simulink model "FINAL_APPROACH_CUSTOM"  (R2020b)
settings: Solver=ode5  StartTime=0.0  StopTime=10  FixedStep=0.01  RelTol=1e-3
values from neighbouring files (symbols this model uses):
  alpha = 0.01    [INPUTS_GRUPPO20.m]
  e_ss = 0.02    [INPUTS_GRUPPO20.m]
  enable_drag = 1    [INPUTS_GRUPPO20.m]
  enable_J2 = 1    [INPUTS_GRUPPO20.m]
  enable_Mgrav = 1    [INPUTS_GRUPPO20.m]
  enable_PD = 1    [INPUTS_GRUPPO20.m]
  enable_SMC = 0    [INPUTS_GRUPPO20.m]
  F_D = -1/2*rho*CD*A*Vx^2    (= -3.88125057814e-05)    [INPUTS_GRUPPO20.m]
  FJ2 = -3*J2*m_c0*mu*r_E^2/(2*r^4)    (= -0.00149705073945)    [INPUTS_GRUPPO20.m]
  gmax = 0.005    [INPUTS_GRUPPO20.m]
  INV_ZZZ = pinv(ZZZ)    [INPUTS_GRUPPO20.m]
  invJ = inv(J)    [INPUTS_GRUPPO20.m]
  Isp1 = 220    [INPUTS_GRUPPO20.m]
  J = J0    [INPUTS_GRUPPO20.m]
  kd = d*eye(3)    [INPUTS_GRUPPO20.m]
  Kd = [1 0.1 1]'    [INPUTS_GRUPPO20.m]
  kf = U_max/edb    (= 10)    [INPUTS_GRUPPO20.m]
  Kp = [0.00001 0.05 0.01]'    [INPUTS_GRUPPO20.m]
  kp1 = k*eye(3)    [INPUTS_GRUPPO20.m]
  Kr = 1    [INPUTS_GRUPPO20.m]
  lambda = 0.03    [INPUTS_GRUPPO20.m]
  m_c0_CUS = m_RB(end)    [INPUTS_GRUPPO20.m]
  omega = (mu/r^3)^0.5    (= 0.00113136572666)    [INPUTS_GRUPPO20.m]
  p_RW = 1    [INPUTS_GRUPPO20.m]
  Pos0 = Pos_RB(end,:)'    [INPUTS_GRUPPO20.m]
  q0_0 = Q_RB(end,1)'    [INPUTS_GRUPPO20.m]
  q_des = [1 0 0 0]'    [INPUTS_GRUPPO20.m]
  qv_0 = Q_RB(end,2:4)'    [INPUTS_GRUPPO20.m]
  tau = -deltaton/log((1-(U_on-U_off)/kf))    [INPUTS_GRUPPO20.m]
  tau_RW = 1.5645e-2    (= 0.015645)    [INPUTS_GRUPPO20.m]
  U_max = 2    [INPUTS_GRUPPO20.m]
  U_off = 0.29    [INPUTS_GRUPPO20.m]
  U_on = 1    [INPUTS_GRUPPO20.m]
  Vel0 = Vel_RB(end,:)'    [INPUTS_GRUPPO20.m]
  wb_0 = wb_RB(end,:)'    [INPUTS_GRUPPO20.m]
  ZZZ = [cos(B)    0      -cos(B)    0 ... (first row only)    [INPUTS_GRUPPO20.m]
undefined symbols (not defined in the file or in its folder): DiscIntNeverNeededParam, magnitude
libraries: vrlib x3, aerolibutil x1, sharedtransform x1
settings Model: Creator=Lucas  LastModifiedBy=Beniamino

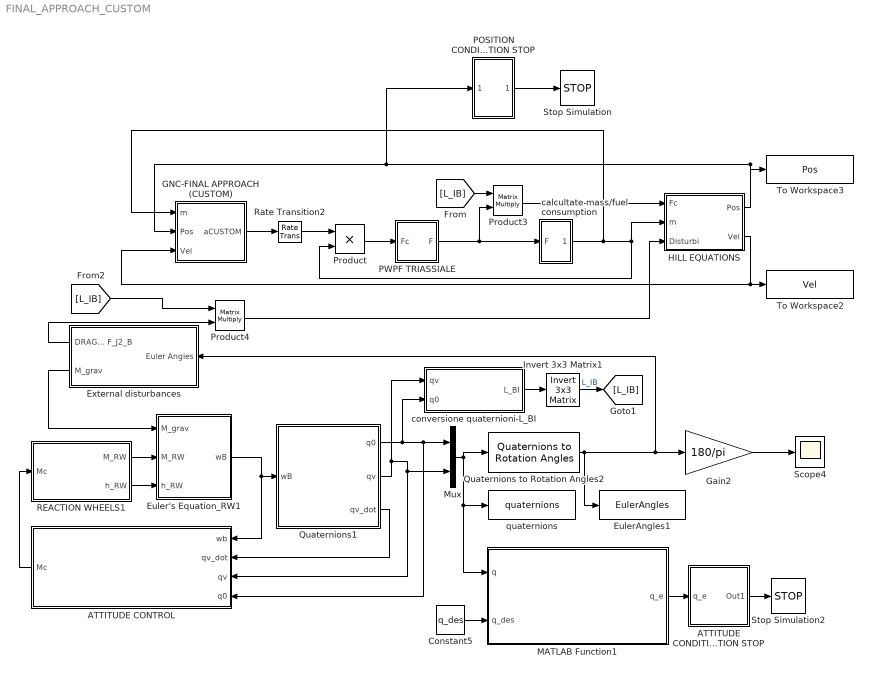
== system FINAL_APPROACH_CUSTOM ==
  ATTITUDE CONDITION SIMULATION STOP : Subsystem
  ATTITUDE CONTROL : Subsystem
  Constant5 : Constant  Value=q_des
  Euler's Equation_RW1 : Subsystem
  EulerAngles1 : ToWorkspace  VariableName=EulerAngles  SampleTime=-1
  External disturbances : Subsystem
  GNC-FINAL APPROACH (CUSTOM) : Subsystem
  Gain2 : Gain  Gain=180/pi
  HILL EQUATIONS : Subsystem
  Invert 3x3 Matrix1 : aerolibutil/Invert  3x3 Matrix
  MATLAB Function1 : MATLAB Function  TreatAsAtomicUnit=on
  Mux : Mux  Inputs=2
  POSITION CONDITION SIMULATION STOP : Subsystem
  PWPF TRIASSIALE : Subsystem
  Product : Product
  Product3 : Product  Multiplication=Matrix(*)
  Product4 : Product  Multiplication=Matrix(*)
  Quaternions to Rotation Angles2 : sharedtransform/Quaternions to Rotation Angles  rotationOrder=ZYX  aMode=aMode
      settings: SourceProductBaseCode=AE,PW,MT,UV,VE,VP
  Quaternions1 : Subsystem
  REACTION WHEELS1 : Subsystem
  Rate Transition2 : RateTransition  OutPortSampleTime=Dt
  Scope4 : Scope
  Stop Simulation : Stop
  Stop Simulation2 : Stop
  To Workspace2 : ToWorkspace  VariableName=Vel  SampleTime=-1
  To Workspace3 : ToWorkspace  VariableName=Pos  SampleTime=-1
  calcultate mass/fuel consumption : Subsystem
  conversione quaternioni-L_BI : Subsystem
  quaternions : ToWorkspace  VariableName=quaternions  SampleTime=-1
  wires:
  GNC-FINAL APPROACH (CUSTOM)/1(aCUSTOM) -> Rate Transition2/1
  Product/1 -> PWPF TRIASSIALE/1(Fc)
  calcultate mass/fuel consumption/1(m) -> GNC-FINAL APPROACH (CUSTOM)/1(m), Product/2, HILL EQUATIONS/2(m)
  Rate Transition2/1 -> Product/1
  PWPF TRIASSIALE/1(F) -> calcultate mass/fuel consumption/1(F), Product3/2
  Product3/1 -> HILL EQUATIONS/1(Fc)
  [L_IB] -> Product3/1
  REACTION WHEELS1/2("h_RW ") -> Euler's Equation_RW1/3(h_RW)
  Quaternions1/1(q0) -> Mux/1, ATTITUDE CONTROL/4(q0), conversione quaternioni-L_BI/2(q0)
  Quaternions1/3(qv_dot) -> ATTITUDE CONTROL/2(qv_dot)
  Gain2/1 -> Scope4/1
  REACTION WHEELS1/1(M_RW) -> Euler's Equation_RW1/2(M_RW)
  External disturbances/2(M_grav) -> Euler's Equation_RW1/1(M_grav)
  conversione quaternioni-L_BI/1(L_BI) -> Invert 3x3 Matrix1/1
  [L_IB] -> Product4/1
  Euler's Equation_RW1/1(wB) -> ATTITUDE CONTROL/1(wb), Quaternions1/1(wB)
  Quaternions to Rotation Angles2/1 -> Gain2/1, External disturbances/1(Euler Angles), EulerAngles1/1
  Constant5/1 -> MATLAB Function1/2(q_des)
  External disturbances/1(DRAG_B + F_J2_B) -> Product4/2
  Mux/1 -> Quaternions to Rotation Angles2/1, MATLAB Function1/1(q), quaternions/1
  ATTITUDE CONTROL/1(Mc) -> REACTION WHEELS1/1(Mc)
  Invert 3x3 Matrix1/1 -> [L_IB]  "L_IB"
  Quaternions1/2(qv) -> ATTITUDE CONTROL/3(qv), Mux/2, conversione quaternioni-L_BI/1(qv)
  Product4/1 -> HILL EQUATIONS/3(Disturbi)
  MATLAB Function1/1(q_e) -> ATTITUDE CONDITION SIMULATION STOP/1(q_e)
  ATTITUDE CONDITION SIMULATION STOP/1(Out1) -> Stop Simulation2/1
  POSITION CONDITION SIMULATION STOP/1(Out1) -> Stop Simulation/1
  HILL EQUATIONS/2(Vel) -> GNC-FINAL APPROACH (CUSTOM)/3(Vel), To Workspace2/1
  HILL EQUATIONS/1(Pos) -> GNC-FINAL APPROACH (CUSTOM)/2(Pos), POSITION CONDITION SIMULATION STOP/1(Pos), To Workspace3/1

== system FINAL_APPROACH_CUSTOM/ATTITUDE CONDITION SIMULATION STOP ==
  q_e : Inport
  Constant2 : Constant
  Constant7 : Constant  Value=0
  Dot Product2 : DotProduct  InputSameDT=on  OutDataTypeStr=Inherit: Inherit via internal rule
  Square Root2 : Sqrt  SaturateOnIntegerOverflow=on
  Subsystem1 : Subsystem
  Switch2 : Switch  Criteria=u2 > Threshold  Threshold=e_ss
  quaternions2 : ToWorkspace  VariableName=normqerr  SampleTime=-1
  Out1 : Outport
  wires:
  Subsystem1/1(q_v_err) -> Dot Product2/1, Dot Product2/2
  Constant7/1 -> Switch2/3
  Dot Product2/1 -> Square Root2/1
  Square Root2/1 -> quaternions2/1, Switch2/2
  Constant2/1 -> Switch2/1
  Switch2/1 -> Out1/1
  q_e/1 -> Subsystem1/1(q_e)

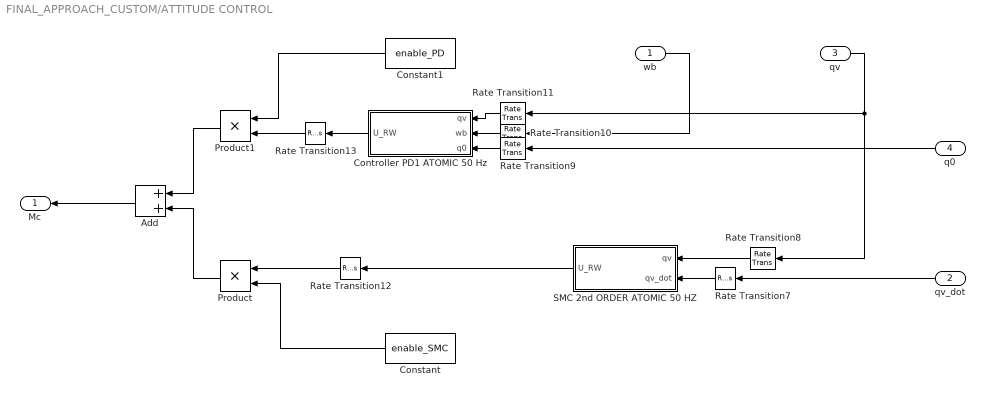
== system FINAL_APPROACH_CUSTOM/ATTITUDE CONTROL ==
  wb : Inport
  qv_dot : Inport  Port=2
  qv : Inport  Port=3
  q0 : Inport  Port=4
  Add : Sum
  Constant : Constant  Value=enable_SMC
  Constant1 : Constant  Value=enable_PD
  Controller PD1 ATOMIC 50 Hz : Subsystem  TreatAsAtomicUnit=on  SystemSampleTime=0.02
  Product : Product
  Product1 : Product
  Rate Transition10 : RateTransition  InitialCondition=wb_0  OutPortSampleTime=Dt_con
  Rate Transition11 : RateTransition  InitialCondition=qv_0  OutPortSampleTime=Dt_con
  Rate Transition12 : RateTransition  OutPortSampleTime=Dt
  Rate Transition13 : RateTransition  OutPortSampleTime=Dt
  Rate Transition7 : RateTransition  InitialCondition=qv_0  OutPortSampleTime=Dt_con
  Rate Transition8 : RateTransition  InitialCondition=q0_0  OutPortSampleTime=Dt_con
  Rate Transition9 : RateTransition  InitialCondition=q0_0  OutPortSampleTime=Dt_con
  SMC 2nd ORDER ATOMIC 50 HZ : Subsystem  TreatAsAtomicUnit=on  SystemSampleTime=0.02
  Mc : Outport
  wires:
  Add/1 -> Mc/1
  qv_dot/1 -> Rate Transition7/1
  q0/1 -> Rate Transition9/1
  SMC 2nd ORDER ATOMIC 50 HZ/1(U_RW) -> Rate Transition12/1
  Controller PD1 ATOMIC 50 Hz/1(U_RW) -> Rate Transition13/1
  Rate Transition8/1 -> SMC 2nd ORDER ATOMIC 50 HZ/1(qv)
  wb/1 -> Rate Transition10/1
  Rate Transition7/1 -> SMC 2nd ORDER ATOMIC 50 HZ/2(qv_dot)
  Rate Transition10/1 -> Controller PD1 ATOMIC 50 Hz/2(wb)
  Rate Transition11/1 -> Controller PD1 ATOMIC 50 Hz/1(qv)
  qv/1 -> Rate Transition11/1, Rate Transition8/1
  Rate Transition9/1 -> Controller PD1 ATOMIC 50 Hz/3(q0)
  Rate Transition12/1 -> Product/1
  Constant/1 -> Product/2
  Rate Transition13/1 -> Product1/2
  Constant1/1 -> Product1/1
  Product1/1 -> Add/1
  Product/1 -> Add/2

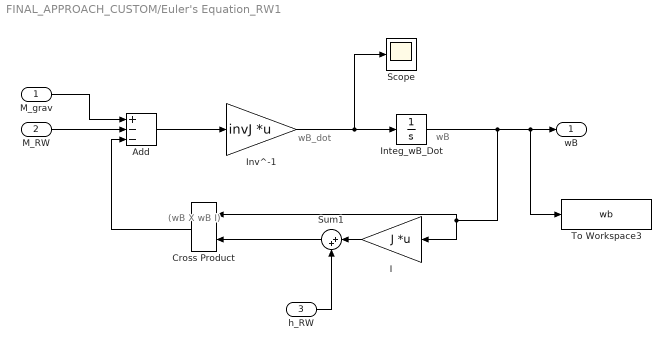
== system FINAL_APPROACH_CUSTOM/Euler's Equation_RW1 ==
  note: (wB X wB I)
  note: wB
  note: wB_dot
  M_grav : Inport
  M_RW : Inport  Port=2
  h_RW : Inport  Port=3
  Add : Sum  Inputs=+--
  Cross Product : vrlib/Utilities/Cross Product
  I : Gain  Gain=J  Multiplication=Matrix(K*u)
  Integ_wB_Dot : Integrator  InitialCondition=wb_0
  Inv^-1 : Gain  Gain=invJ  Multiplication=Matrix(K*u)
  Scope : Scope
  Sum1 : Sum  Inputs=|++
  To Workspace3 : ToWorkspace  VariableName=wb  SampleTime=-1
  wB : Outport  VectorParamsAs1DForOutWhenUnconnected=off
  wires:
  M_grav/1 -> Add/1
  Sum1/1 -> Cross Product/2
  h_RW/1 -> Sum1/2
  Integ_wB_Dot/1 -> To Workspace3/1, wB/1, Cross Product/1, I/1
  I/1 -> Sum1/1
  M_RW/1 -> Add/2
  Add/1 -> Inv^-1/1
  Inv^-1/1 -> Scope/1, Integ_wB_Dot/1
  Cross Product/1 -> Add/3

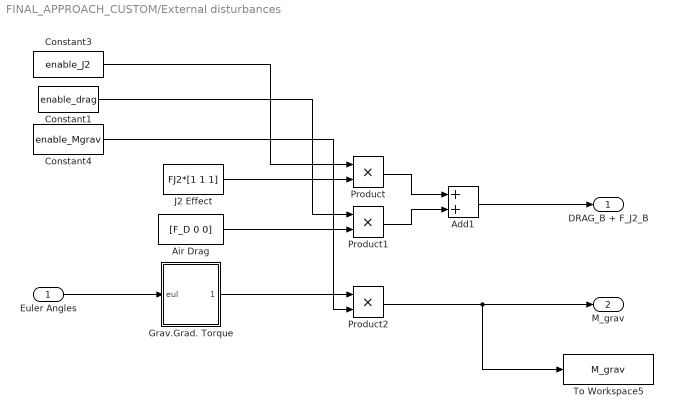
== system FINAL_APPROACH_CUSTOM/External disturbances ==
  Euler Angles : Inport
  Add1 : Sum
  Air Drag : Constant  Value=[F_D 0 0]
  Constant1 : Constant  Value=enable_drag
  Constant3 : Constant  Value=enable_J2
  Constant4 : Constant  Value=enable_Mgrav
  Grav.Grad. Torque : Subsystem
  J2 Effect : Constant  Value=FJ2*[1 1 1]
  Product : Product
  Product1 : Product
  Product2 : Product
  To Workspace5 : ToWorkspace  VariableName=M_grav  SampleTime=-1
  DRAG_B + F_J2_B : Outport
  M_grav : Outport  Port=2
  wires:
  Grav.Grad. Torque/1(M_grav) -> Product2/1
  Euler Angles/1 -> Grav.Grad. Torque/1(eul)
  Add1/1 -> DRAG_B + F_J2_B/1
  Constant3/1 -> Product/1
  J2 Effect/1 -> Product/2
  Constant1/1 -> Product1/1
  Air Drag/1 -> Product1/2
  Constant4/1 -> Product2/2
  Product/1 -> Add1/1
  Product1/1 -> Add1/2
  Product2/1 -> To Workspace5/1, M_grav/1

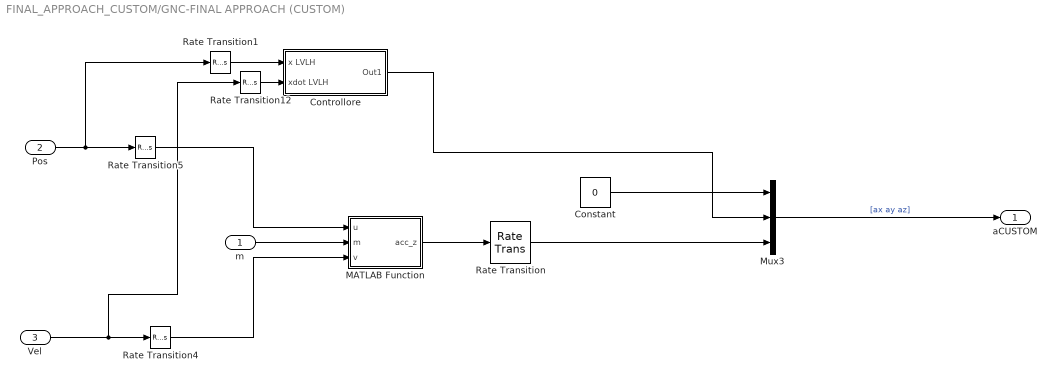
== system FINAL_APPROACH_CUSTOM/GNC-FINAL APPROACH (CUSTOM) ==
  m : Inport
  Pos : Inport  Port=2
  Vel : Inport  Port=3
  Constant : Constant  Value=0
  Controllore : Subsystem
  MATLAB Function : MATLAB Function  TreatAsAtomicUnit=on
  Mux3 : Mux  Inputs=3
  Rate Transition : RateTransition  OutPortSampleTime=Dt_con
  Rate Transition1 : RateTransition  InitialCondition=Pos0  OutPortSampleTime=Dt_con
  Rate Transition12 : RateTransition  InitialCondition=Vel0  OutPortSampleTime=Dt_con
  Rate Transition4 : RateTransition  InitialCondition=Vel0  OutPortSampleTime=Dt_guid
  Rate Transition5 : RateTransition  InitialCondition=Pos0  OutPortSampleTime=Dt_guid
  aCUSTOM : Outport
  wires:
  Rate Transition1/1 -> Controllore/1(x LVLH)
  Rate Transition12/1 -> Controllore/2(xdot LVLH)
  MATLAB Function/1(acc_z) -> Rate Transition/1
  Constant/1 -> Mux3/1
  Mux3/1 -> aCUSTOM/1  "[ax ay az]"
  Pos/1 -> Rate Transition5/1, Rate Transition1/1
  Controllore/1(Out1) -> Mux3/2
  Vel/1 -> Rate Transition12/1, Rate Transition4/1
  Rate Transition5/1 -> MATLAB Function/1(u)
  Rate Transition4/1 -> MATLAB Function/3(v)
  m/1 -> MATLAB Function/2(m)
  Rate Transition/1 -> Mux3/3

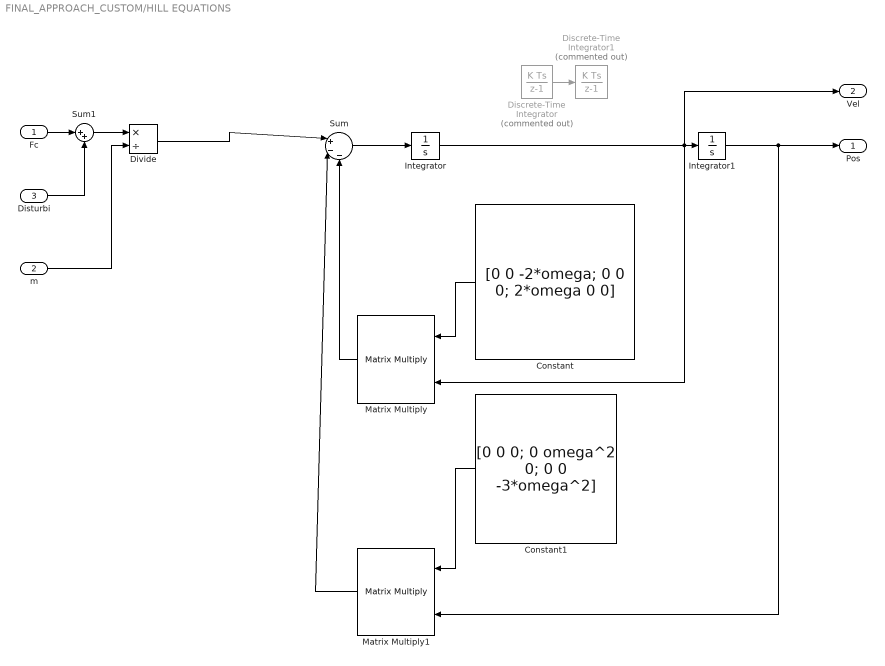
== system FINAL_APPROACH_CUSTOM/HILL EQUATIONS ==
  Fc : Inport
  m : Inport  Port=2
  Disturbi : Inport  Port=3
  Constant : Constant  Value=[0 0 -2*omega; 0 0 0; 2*omega 0 0]
  Constant1 : Constant  Value=[0 0 0; 0 omega^2 0; 0 0 -3*omega^2]
  Discrete-Time Integrator : DiscreteIntegrator  Commented=on  InitialCondition=Vel0  SampleTime=-1  ICPrevOutput=DiscIntNeverNeededParam  ICPrevScaledInput=DiscIntNeverNeededParam
  Discrete-Time Integrator1 : DiscreteIntegrator  Commented=on  InitialCondition=Pos0  SampleTime=-1  ICPrevOutput=DiscIntNeverNeededParam  ICPrevScaledInput=DiscIntNeverNeededParam
  Divide : Product  Inputs=*/
  Integrator : Integrator  InitialCondition=Vel0
  Integrator1 : Integrator  InitialCondition=Pos0
  Matrix Multiply : Product  Multiplication=Matrix(*)
  Matrix Multiply1 : Product  Multiplication=Matrix(*)
  Sum : Sum  Inputs=|+--
  Sum1 : Sum  Inputs=|++
  Pos : Outport
  Vel : Outport  Port=2
  wires:
  Constant/1 -> Matrix Multiply/1
  Sum1/1 -> Divide/1
  Disturbi/1 -> Sum1/2
  Integrator/1 -> Integrator1/1, Vel/1, Matrix Multiply/2
  Fc/1 -> Sum1/1
  m/1 -> Divide/2
  Matrix Multiply1/1 -> Sum/2
  Matrix Multiply/1 -> Sum/3
  Constant1/1 -> Matrix Multiply1/1
  Integrator1/1 -> Matrix Multiply1/2, Pos/1
  Sum/1 -> Integrator/1
  Divide/1 -> Sum/1
  Discrete-Time Integrator/1 -> Discrete-Time Integrator1/1

== system FINAL_APPROACH_CUSTOM/POSITION CONDITION SIMULATION STOP ==
  Pos : Inport
  Constant : Constant
  Constant1 : Constant  Value=0
  Demux2 : Demux  Outputs=3
  Switch : Switch  Criteria=u2 > Threshold  Threshold=-2
  Terminator3 : Terminator
  Terminator4 : Terminator
  Out1 : Outport
  wires:
  Demux2/2 -> Terminator4/1
  Constant1/1 -> Switch/3
  Constant/1 -> Switch/1
  Demux2/1 -> Switch/2
  Switch/1 -> Out1/1
  Pos/1 -> Demux2/1
  Demux2/3 -> Terminator3/1

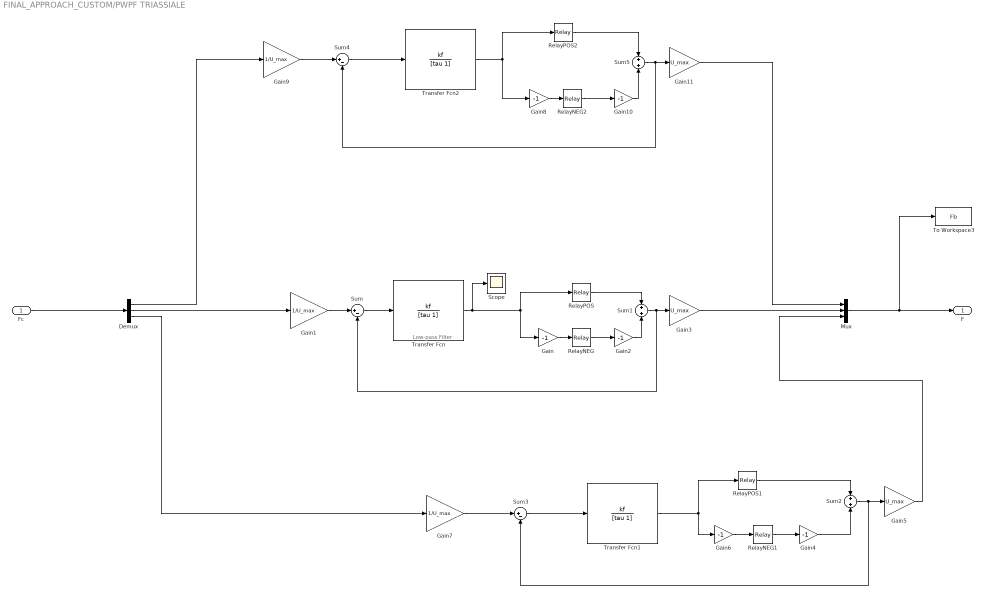
== system FINAL_APPROACH_CUSTOM/PWPF TRIASSIALE ==
  note: Low-pass Filter
  Fc : Inport
  Demux : Demux  Outputs=3
  Gain{,2,4,6,8,10} (6 alike) : Gain  Gain=-1
  Gain1 : Gain  Gain=1/U_max
  Gain11 : Gain  Gain=U_max
  Gain3 : Gain  Gain=U_max
  Gain5 : Gain  Gain=U_max
  Gain7 : Gain  Gain=1/U_max
  Gain9 : Gain  Gain=1/U_max
  Mux : Mux  Inputs=3
  RelayNEG : Relay  OnSwitchValue=U_on  OffSwitchValue=U_off
  RelayNEG1 : Relay  OnSwitchValue=U_on  OffSwitchValue=U_off
  RelayNEG2 : Relay  OnSwitchValue=U_on  OffSwitchValue=U_off
  RelayPOS : Relay  OnSwitchValue=U_on  OffSwitchValue=U_off
  RelayPOS1 : Relay  OnSwitchValue=U_on  OffSwitchValue=U_off
  RelayPOS2 : Relay  OnSwitchValue=U_on  OffSwitchValue=U_off
  Scope : Scope
  Sum : Sum  Inputs=|+-
  Sum1 : Sum  Inputs=+|+
  Sum2 : Sum  Inputs=+|+
  Sum3 : Sum  Inputs=|+-
  Sum4 : Sum  Inputs=|+-
  Sum5 : Sum  Inputs=+|+
  To Workspace3 : ToWorkspace  VariableName=Fb  SampleTime=-1
  Transfer Fcn : TransferFcn  Numerator=kf  Denominator=[tau 1]
  Transfer Fcn1 : TransferFcn  Numerator=kf  Denominator=[tau 1]
  Transfer Fcn2 : TransferFcn  Numerator=kf  Denominator=[tau 1]
  F : Outport  VectorParamsAs1DForOutWhenUnconnected=off
  wires:
  Fc/1 -> Demux/1
  Transfer Fcn/1 -> Gain/1, RelayPOS/1, Scope/1
  Gain/1 -> RelayNEG/1
  RelayPOS/1 -> Sum1/1
  RelayNEG/1 -> Gain2/1
  Sum1/1 -> Sum/2, Gain3/1
  Gain1/1 -> Sum/1
  Sum/1 -> Transfer Fcn/1
  Gain2/1 -> Sum1/2
  Transfer Fcn1/1 -> Gain6/1, RelayPOS1/1
  Gain6/1 -> RelayNEG1/1
  RelayNEG1/1 -> Gain4/1
  RelayPOS1/1 -> Sum2/1
  Gain4/1 -> Sum2/2
  Sum2/1 -> Sum3/2, Gain5/1
  Sum3/1 -> Transfer Fcn1/1
  Gain7/1 -> Sum3/1
  Demux/3 -> Gain7/1
  Demux/2 -> Gain1/1
  Demux/1 -> Gain9/1
  Gain9/1 -> Sum4/1
  Sum4/1 -> Transfer Fcn2/1
  RelayNEG2/1 -> Gain10/1
  Gain8/1 -> RelayNEG2/1
  Transfer Fcn2/1 -> Gain8/1, RelayPOS2/1
  Gain10/1 -> Sum5/2
  RelayPOS2/1 -> Sum5/1
  Sum5/1 -> Sum4/2, Gain11/1
  Mux/1 -> To Workspace3/1, F/1
  Gain3/1 -> Mux/2
  Gain5/1 -> Mux/3
  Gain11/1 -> Mux/1

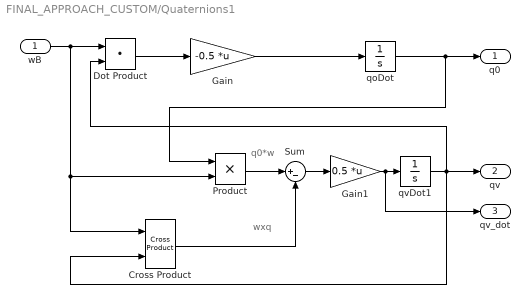
== system FINAL_APPROACH_CUSTOM/Quaternions1 ==
  note: wxq
  note: q0*w
  wB : Inport
  Cross Product : vrlib/Utilities/Cross Product
  Dot Product : DotProduct  InputSameDT=on  OutDataTypeStr=Inherit: Inherit via internal rule
  Gain : Gain  Gain=-0.5  Multiplication=Matrix(K*u)
  Gain1 : Gain  Gain=0.5  Multiplication=Matrix(K*u)
  Product : Product  RndMeth=Zero
  Sum : Sum  Inputs=|+-
  qoDot : Integrator  InitialCondition=q0_0
  qvDot1 : Integrator  InitialCondition=qv_0
  q0 : Outport  VectorParamsAs1DForOutWhenUnconnected=off
  qv : Outport  Port=2  VectorParamsAs1DForOutWhenUnconnected=off
  qv_dot : Outport  Port=3  VectorParamsAs1DForOutWhenUnconnected=off
  wires:
  qoDot/1 -> q0/1, Product/1
  qvDot1/1 -> Cross Product/2, qv/1, Dot Product/2
  wB/1 -> Cross Product/1, Product/2, Dot Product/1
  Dot Product/1 -> Gain/1
  Gain/1 -> qoDot/1
  Product/1 -> Sum/1
  Cross Product/1 -> Sum/2
  Sum/1 -> Gain1/1
  Gain1/1 -> qvDot1/1, qv_dot/1

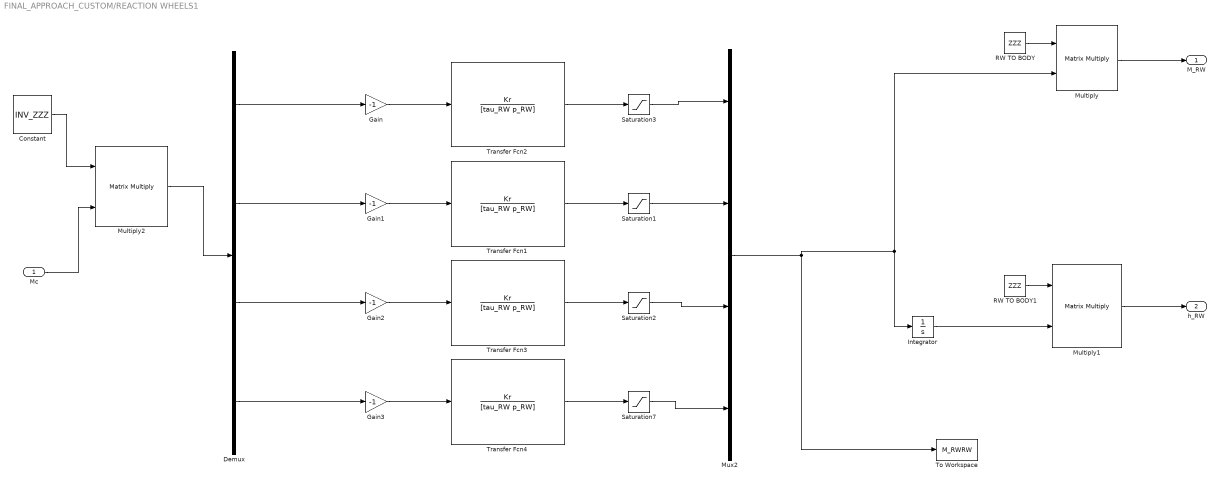
== system FINAL_APPROACH_CUSTOM/REACTION WHEELS1 ==
  Mc : Inport
  Constant : Constant  Value=INV_ZZZ
  Demux : Demux
  Gain{,1..3} (4 alike) : Gain  Gain=-1
  Integrator : Integrator
  Multiply : Product  Multiplication=Matrix(*)
  Multiply1 : Product  Multiplication=Matrix(*)
  Multiply2 : Product  Multiplication=Matrix(*)
  Mux2 : Mux
  RW TO BODY : Constant  Value=ZZZ
  RW TO BODY1 : Constant  Value=ZZZ
  Saturation{1..3,7} (4 alike) : Saturate  UpperLimit=gmax  LowerLimit=-gmax
  To Workspace : ToWorkspace  VariableName=M_RWRW  SampleTime=-1
  Transfer Fcn{1..4} (4 alike) : TransferFcn  Numerator=Kr  Denominator=[tau_RW p_RW]
  M_RW : Outport  VectorParamsAs1DForOutWhenUnconnected=off
  "h_RW " : Outport  Port=2  VectorParamsAs1DForOutWhenUnconnected=off
  wires:
  Mc/1 -> Multiply2/2
  Multiply/1 -> M_RW/1
  Demux/1 -> Gain/1
  Demux/2 -> Gain1/1
  Demux/3 -> Gain2/1
  Gain/1 -> Transfer Fcn2/1
  Gain1/1 -> Transfer Fcn1/1
  Gain2/1 -> Transfer Fcn3/1
  Multiply1/1 -> "h_RW "/1
  Demux/4 -> Gain3/1
  Gain3/1 -> Transfer Fcn4/1
  RW TO BODY/1 -> Multiply/1
  RW TO BODY1/1 -> Multiply1/1
  Constant/1 -> Multiply2/1
  Multiply2/1 -> Demux/1
  Transfer Fcn4/1 -> Saturation7/1
  Mux2/1 -> To Workspace/1, Multiply/2, Integrator/1
  Integrator/1 -> Multiply1/2
  Saturation7/1 -> Mux2/4
  Transfer Fcn3/1 -> Saturation2/1
  Saturation2/1 -> Mux2/3
  Transfer Fcn1/1 -> Saturation1/1
  Saturation1/1 -> Mux2/2
  Transfer Fcn2/1 -> Saturation3/1
  Saturation3/1 -> Mux2/1

== system FINAL_APPROACH_CUSTOM/calcultate mass//fuel consumption ==
  F : Inport
  Add : Sum  Inputs=+-
  Constant : Constant  Value=m_c0_CUS
  Dot Product : DotProduct  InputSameDT=on  OutDataTypeStr=Inherit: Inherit via internal rule
  Gain : Gain  Gain=1/(Isp1*9.81)
  Integrator : Integrator
  Sqrt : Sqrt  SaturateOnIntegerOverflow=on
  To Workspace1 : ToWorkspace  VariableName=m  SampleTime=-1
  To Workspace4 : ToWorkspace  VariableName=mf  SampleTime=-1
  m : Outport
  wires:
  F/1 -> Dot Product/2, Dot Product/1
  Dot Product/1 -> Sqrt/1
  Sqrt/1 -> Gain/1
  Gain/1 -> Integrator/1  "m_dot"
  Constant/1 -> Add/1
  Add/1 -> To Workspace1/1, m/1
  Integrator/1 -> To Workspace4/1, Add/2

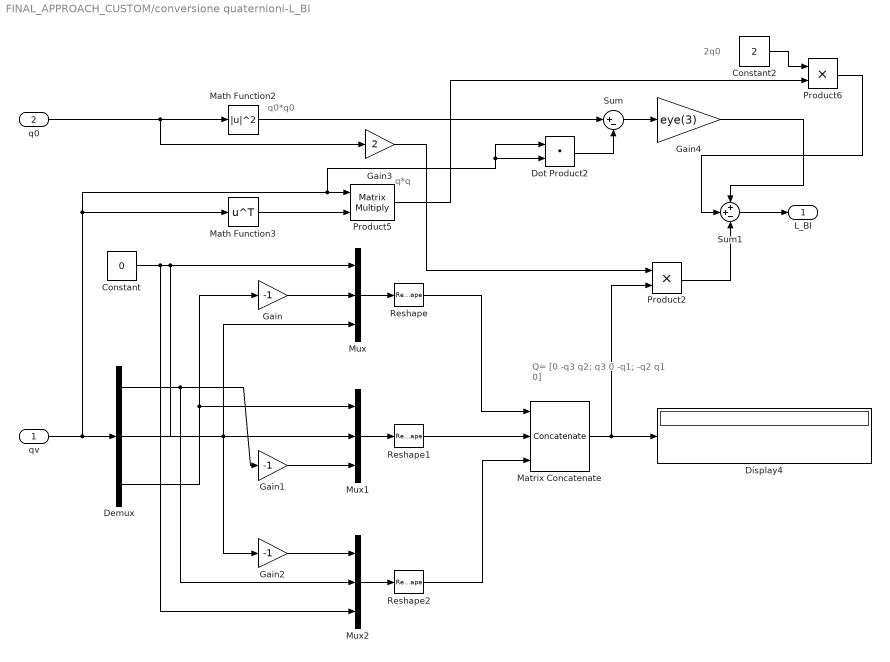
== system FINAL_APPROACH_CUSTOM/conversione quaternioni-L_BI ==
  note: Q= [0 -q3 q2;
      | 	q3 0 -q1;
      | 	-q2 q1 0]
  note: 2q0
  note: q*q
  note: q0*q0
  qv : Inport
  q0 : Inport  Port=2
  Constant : Constant  Value=0
  Constant2 : Constant  Value=2
  Demux : Demux  Outputs=3
  Display4 : Display
  Dot Product2 : DotProduct  InputSameDT=on  OutDataTypeStr=Inherit: Inherit via internal rule
  Gain : Gain  Gain=-1
  Gain1 : Gain  Gain=-1
  Gain2 : Gain  Gain=-1
  Gain3 : Gain  Gain=2
  Gain4 : Gain  Gain=eye(3)
  Math Function2 : Math  Operator=magnitude^2  SignedPower=on  SaturateOnIntegerOverflow=on
  Math Function3 : Math  Operator=transpose  SignedPower=on  SaturateOnIntegerOverflow=on
  Matrix Concatenate : Concatenate  NumInputs=3  Mode=Multidimensional array
  Mux : Mux  Inputs=3
  Mux1 : Mux  Inputs=3
  Mux2 : Mux  Inputs=3
  Product2 : Product  RndMeth=Zero
  Product5 : Product  Multiplication=Matrix(*)
  Product6 : Product
  Reshape : Reshape  OutputDimensionality=Row vector (2-D)
  Reshape1 : Reshape  OutputDimensionality=Row vector (2-D)
  Reshape2 : Reshape  OutputDimensionality=Row vector (2-D)
  Sum : Sum  Inputs=|+-
  Sum1 : Sum  Inputs=++-
  L_BI : Outport  VectorParamsAs1DForOutWhenUnconnected=off
  wires:
  qv/1 -> Demux/1, Product5/1, Dot Product2/2, Dot Product2/1, Math Function3/1
  Constant/1 -> Mux/1, Mux1/2, Mux2/3
  Demux/3 -> Gain/1, Mux1/1
  Gain/1 -> Mux/2
  Demux/2 -> Mux/3, Gain2/1
  Gain1/1 -> Mux1/3
  Demux/1 -> Gain1/1, Mux2/2
  Gain2/1 -> Mux2/1
  q0/1 -> Gain3/1, Math Function2/1
  Math Function2/1 -> Sum/1
  Gain4/1 -> Sum1/1
  Product6/1 -> Sum1/2
  Product2/1 -> Sum1/3
  Sum1/1 -> L_BI/1
  Matrix Concatenate/1 -> Product2/2, Display4/1
  Mux/1 -> Reshape/1
  Reshape/1 -> Matrix Concatenate/1
  Mux2/1 -> Reshape2/1
  Reshape2/1 -> Matrix Concatenate/3
  Mux1/1 -> Reshape1/1
  Reshape1/1 -> Matrix Concatenate/2
  Sum/1 -> Gain4/1
  Math Function3/1 -> Product5/2
  Gain3/1 -> Product2/1
  Product5/1 -> Product6/2
  Constant2/1 -> Product6/1
  Dot Product2/1 -> Sum/2

== system FINAL_APPROACH_CUSTOM/ATTITUDE CONDITION SIMULATION STOP/Subsystem1 ==
  q_e : Inport
  Demux : Demux
  Mux1 : Mux  Inputs=3
  Terminator : Terminator
  q_v_err : Outport  VectorParamsAs1DForOutWhenUnconnected=off
  wires:
  Demux/3 -> Mux1/2
  Demux/2 -> Mux1/1
  Demux/4 -> Mux1/3
  Demux/1 -> Terminator/1
  q_e/1 -> Demux/1
  Mux1/1 -> q_v_err/1

== system FINAL_APPROACH_CUSTOM/ATTITUDE CONTROL/Controller PD1 ATOMIC 50 Hz ==
  qv : Inport
  wb : Inport  Port=2
  q0 : Inport  Port=3
  Constant : Constant  Value=kp1
  Gain : Gain  Gain=kd  Multiplication=Matrix(K*u) (u vector)
  Multiply : Product  Multiplication=Matrix(*)
  Multiply1 : Product
  Sign : Signum
  Sum : Sum  Inputs=|--
  U_RW : Outport  VectorParamsAs1DForOutWhenUnconnected=off
  wires:
  Gain/1 -> Sum/1
  Constant/1 -> Multiply/1
  q0/1 -> Sign/1
  Multiply/1 -> Multiply1/1
  wb/1 -> Gain/1
  Sign/1 -> Multiply1/2
  Multiply1/1 -> Sum/2
  Sum/1 -> U_RW/1
  qv/1 -> Multiply/2

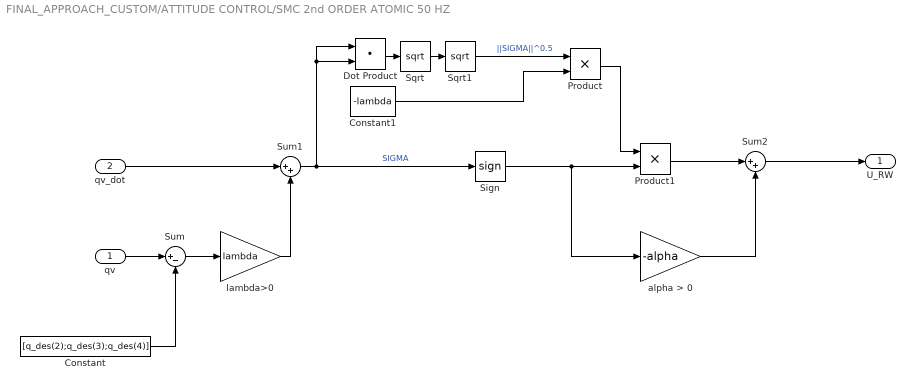
== system FINAL_APPROACH_CUSTOM/ATTITUDE CONTROL/SMC 2nd ORDER ATOMIC 50 HZ ==
  qv : Inport
  qv_dot : Inport  Port=2
  Constant : Constant  Value=[q_des(2);q_des(3);q_des(4)]
  Constant1 : Constant  Value=-lambda
  Dot Product : DotProduct  InputSameDT=on  OutDataTypeStr=Inherit: Inherit via internal rule
  Product : Product
  Product1 : Product
  Sign : Signum
  Sqrt : Sqrt  SaturateOnIntegerOverflow=on
  Sqrt1 : Sqrt  SaturateOnIntegerOverflow=on
  Sum : Sum  Inputs=|+-
  Sum1 : Sum  Inputs=|++
  Sum2 : Sum  Inputs=|++
  alpha > 0 : Gain  Gain=-alpha
  lambda>0 : Gain  Gain=lambda
  U_RW : Outport
  wires:
  Constant1/1 -> Product/2
  alpha > 0/1 -> Sum2/2
  Product1/1 -> Sum2/1
  Dot Product/1 -> Sqrt/1
  Sum/1 -> lambda>0/1
  Sum2/1 -> U_RW/1
  Product/1 -> Product1/1
  Sign/1 -> alpha > 0/1, Product1/2
  lambda>0/1 -> Sum1/2
  Constant/1 -> Sum/2
  Sum1/1 -> Sign/1, Dot Product/1, Dot Product/2  "SIGMA"
  Sqrt/1 -> Sqrt1/1
  Sqrt1/1 -> Product/1  "||SIGMA||^0.5"
  qv_dot/1 -> Sum1/1
  qv/1 -> Sum/1

== system FINAL_APPROACH_CUSTOM/External disturbances/Grav.Grad. Torque ==
  eul : Inport
  Constant3 : Constant  Value=J
  Constant4 : Constant  Value=3*omega^2
  Cross Product : vrlib/Utilities/Cross Product
  MATLAB function : MATLAB Function  TreatAsAtomicUnit=on
  Matrix Multiply : Product  Multiplication=Matrix(*)
  Product2 : Product
  M_grav : Outport
  wires:
  Constant3/1 -> Matrix Multiply/1
  MATLAB function/1(r) -> Matrix Multiply/2, Cross Product/1
  Cross Product/1 -> Product2/2
  Constant4/1 -> Product2/1
  Product2/1 -> M_grav/1
  eul/1 -> MATLAB function/1(eul)
  Matrix Multiply/1 -> Cross Product/2

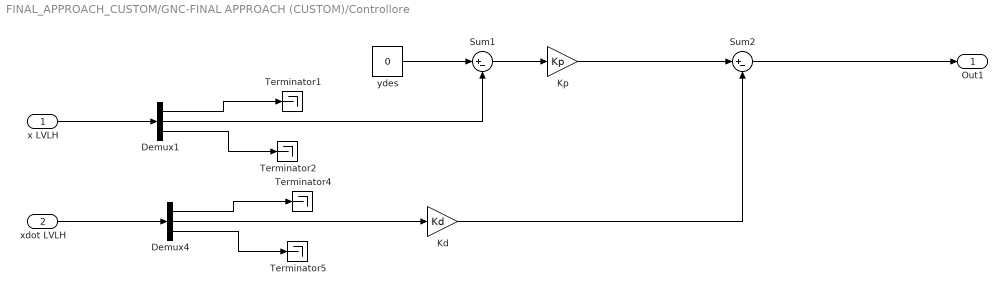
== system FINAL_APPROACH_CUSTOM/GNC-FINAL APPROACH (CUSTOM)/Controllore ==
  x LVLH : Inport
  xdot LVLH : Inport  Port=2
  Demux1 : Demux  Outputs=3
  Demux4 : Demux  Outputs=3
  Kd : Gain  Gain=Kd
  Kp : Gain  Gain=Kp
  Sum1 : Sum  Inputs=|+-
  Sum2 : Sum  Inputs=|+-
  Terminator{1..2,4..5} (4 alike) : Terminator
  ydes : Constant  Value=0
  Out1 : Outport
  wires:
  Demux4/2 -> Kd/1
  Demux4/1 -> Terminator4/1
  Demux4/3 -> Terminator5/1
  xdot LVLH/1 -> Demux4/1
  Demux1/1 -> Terminator1/1
  Demux1/3 -> Terminator2/1
  Demux1/2 -> Sum1/2
  x LVLH/1 -> Demux1/1
  ydes/1 -> Sum1/1
  Sum1/1 -> Kp/1
  Kd/1 -> Sum2/2
  Kp/1 -> Sum2/1
  Sum2/1 -> Out1/1

== matlab function FINAL_APPROACH_CUSTOM/External disturbances/Grav.Grad. Torque/MATLAB function ==
  data: eul input; r output
function r = fcn(eul)
    r = [-sin(eul(2)); sin(eul(3)); 1-(sin(eul(2)))^2-(sin(eul(3)))^2];

== matlab function FINAL_APPROACH_CUSTOM/MATLAB Function1 ==
  data: q input; q_e output; q_des input
function q_e = quaternion_error(q, q_des)
%#codegen

q_inv = [q_des(1) -q_des(2) -q_des(3) -q_des(4)]'/(q_des(1)^2+q_des(2)^2 + q_des(3)^2+q_des(4)^2);

Q   = [q_inv(1) -q_inv(2) -q_inv(3) -q_inv(4)
       q_inv(2)  q_inv(1) -q_inv(4)  q_inv(3)
       q_inv(3)  q_inv(4)  q_inv(1) -q_inv(2)
       q_inv(4) -q_inv(3)  q_inv(2)  q_inv(1)];
q_e =Q*q;

== matlab function FINAL_APPROACH_CUSTOM/GNC-FINAL APPROACH (CUSTOM)/MATLAB Function ==
  data: u input; m input; v input; acc_z output
function acc_z=fcn(u,m,v)
acc_z=0;
Fthr=2;
omega=0.0011;
Vx=v(1);
Vz=v(3);
x=u(1);
z=u(3);
posizione_cono=(-0.9/498)*x+0.0964;
if x<-250
    precisione=0.2;
    forza=0.5;
else
    if x<-50
        precisione=0.2;
        forza=0.35;
    else
        precisione=0.05;
        forza=0.2;
    end
end

if abs(z)>=(posizione_cono*precisione)
     if sign(Vz)==sign(z)
        acc_z=-forza*sign(z)*Fthr/m;
     end
end
